simulink model "main_model"  (R2015a)
settings: Solver=ode3  StartTime=0.0  StopTime=30  FixedStep=Ts  RelTol=1e-3
settings Model: Creator=chris  LastModifiedBy=chris

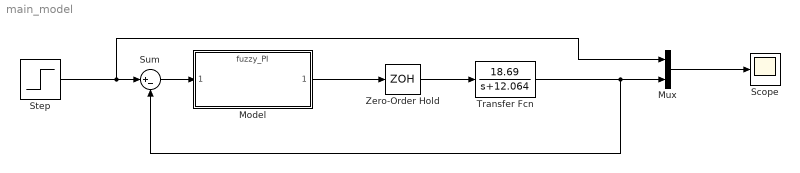
== system main_model ==
  Model : ModelReference  ModelNameDialog=fuzzy_PI.slx  SimulationMode=Normal  ModelReferenceVersion=1.14  CopyOfModelName=fuzzy_PI.slx  DefaultDataLogging=on
  Mux : Mux  Inputs=2
  Scope : Scope
      settings: TimeRange=30  YMin=-20  YMax=160
  Step : Step  After=150
  Sum : Sum  Inputs=|+-
  Transfer Fcn : TransferFcn  Numerator=[18.69]  Denominator=[1 12.064]
  Zero-Order Hold : ZeroOrderHold  SampleTime=-1
  wires:
  Step/1 -> Mux/1, Sum/1
  Sum/1 -> Model/1
  Model/1 -> Zero-Order Hold/1
  Zero-Order Hold/1 -> Transfer Fcn/1
  Transfer Fcn/1 -> Mux/2, Sum/2
  Mux/1 -> Scope/1
